simulink library "LibraryFM"  (R2016b)
settings: Solver=VariableStepAuto  StartTime=0.0  StopTime=10.0  RelTol=1e-3
undefined symbols (not defined in the file or in its folder): ActuatorStruct, drivePeakCurrent, FM1, Lb, Lf, Lu, motorTorqueConstant, RobotStruct, sampleTime, transmissionRatio
undefined symbols (not defined in the file): JointAbsoluteEncoderCounts_rev
libraries: simulink x34, LibraryFM x13, VariousBlocksLibrary x4, dspstat3 x1, simulink_extras x1, FM_Library x1
(part 1 of 3)
settings Model: Creator=niekbeckers  LastModifiedBy=Labuser

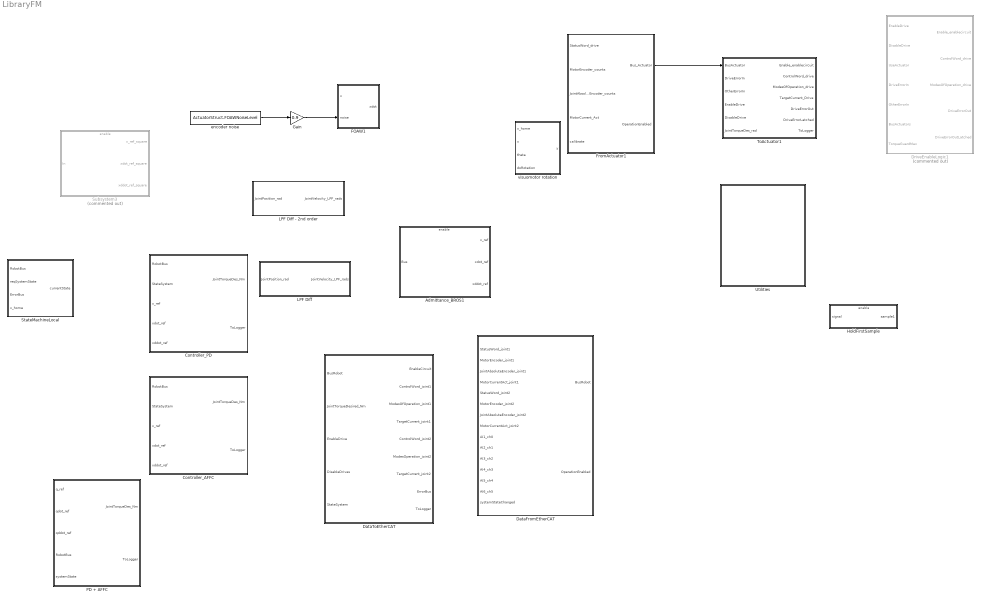
== system LibraryFM ==
  Admittance_BROS1 : Subsystem
  Controller_AFFC : Subsystem
  Controller_PD : Subsystem
  DataFromEtherCAT : Subsystem
  DataToEtherCAT : Subsystem
  DriveEnableLogic1 : Subsystem  Commented=on
  FOAW1 : MATLAB Function  TreatAsAtomicUnit=on
  FromActuator1 : Subsystem  mask{ActuatorStruct=RobotStruct.Actuator1}
      mask prompts: ActuatorStruct "Actuator Struct"
  Gain : Gain  Gain=0.9
  HoldFirstSample : Subsystem
  LPF Diff : Subsystem
  LPF Diff - 2nd order : Subsystem
  PD + AFFC : Subsystem  AncestorBlock=LibraryFM/Robot1/Controller/PD + Nonlinear ID
  StateMachineLocal : Subsystem
  Subsystem3 : Subsystem  Commented=on
  ToActuator1 : Subsystem  mask{ActuatorStruct=RobotStruct.Actuator1}
      mask prompts: ActuatorStruct "Actuator Struct"
  Utilities : Subsystem
  encoder noise : Constant  Value=ActuatorStruct.FOAWNoiseLevel
  visuomotor rotation : MATLAB Function  TreatAsAtomicUnit=on
  wires:
  FromActuator1/1(Bus_Actuator) -> ToActuator1/1(BusActuator)
  Gain/1 -> FOAW1/2(noise)
  encoder noise/1 -> Gain/1

== system LibraryFM/Admittance_BROS1 ==
  Bus : Inport
  Enable : EnablePort  StatesWhenEnabling=reset
  Bus Selector : BusSelector  OutputSignals=BusFTSensor.FxFyOpSpace
  Bus Selector1 : BusSelector  OutputSignals=xOpSpace.x_AbsEnc
  Constant : Constant
  HoldFirstSampleOnEnable : Subsystem
  Sum : Sum  Inputs=++|
  Terminator : Terminator
  Terminator1 : Terminator
  Terminator2 : Terminator
  Virtual model : MATLAB Function  TreatAsAtomicUnit=on
  virtual damping : Constant  Value=0.05
  virtual mass : Constant  Value=0.5
  x_prev : UnitDelay  SampleTime=-1
  xdot_prev : UnitDelay  SampleTime=-1
  x_ref : Outport
  xdot_ref : Outport  Port=2
  xddot_ref : Outport  Port=3
  wires:
  Virtual model/1(lim_pos) -> Terminator/1
  virtual damping/1 -> Virtual model/2(B_v)
  Sum/1 -> x_ref/1
  Virtual model/6(xddot1) -> xddot_ref/1
  x_prev/1 -> Virtual model/4(x1_prev)
  xdot_prev/1 -> Virtual model/5(xdot1_prev)
  Virtual model/5(xdot1) -> xdot_prev/1, xdot_ref/1
  Virtual model/4(x1) -> Sum/2, x_prev/1
  virtual mass/1 -> Virtual model/1(M_v)
  Virtual model/2(lim_vel) -> Terminator1/1
  Virtual model/3(lim_acc) -> Terminator2/1
  Bus/1 -> Bus Selector1/1, Bus Selector/1
  Bus Selector/1 -> Virtual model/3(F)  "<FxFyOpSpace>"
  Constant/1 -> HoldFirstSampleOnEnable/Enable
  Bus Selector1/1 -> HoldFirstSampleOnEnable/1(x)  "<x_AbsEnc>"
  HoldFirstSampleOnEnable/1(x0) -> Sum/1

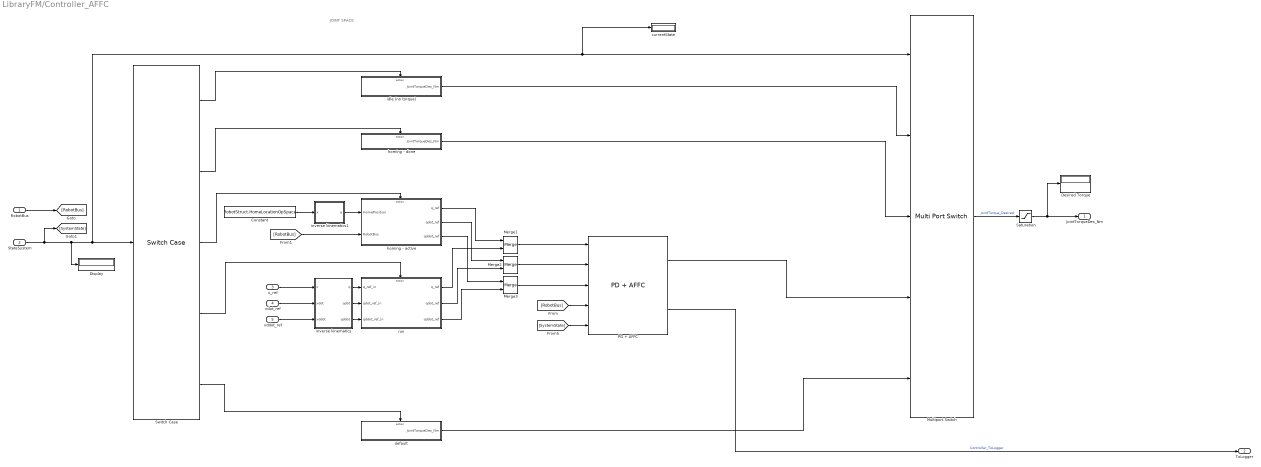
== system LibraryFM/Controller_AFFC ==
  note: JOINT SPACE
  RobotBus : Inport
  StateSystem : Inport  Port=2
  x_ref : Inport  Port=3
  xdot_ref : Inport  Port=4
  xddot_ref : Inport  Port=5
  Constant : Constant  Value=RobotStruct.HomeLocationOpSpace
  Desired Torque : Display
  Display : Display
  Merge1 : Merge  InitialOutput=[0;0]
  Merge2 : Merge  InitialOutput=[0;0]
  Merge3 : Merge  InitialOutput=[0;0]
  Multiport Switch : MultiPortSwitch  DataPortOrder=Specify indices  Inputs=4  DataPortIndices={[0,1,2,201,299,301],[399],[302,4]}  DataPortForDefault=Additional data port
  PD + AFFC : LibraryFM/PD + AFFC
  Saturation : Saturate  UpperLimit=1  LowerLimit=-2
  Switch Case : SwitchCase  CaseConditions={[0,1,2,201,299,301],[399],[302],[4]}
  currentState : Display
  default : Subsystem  TreatAsAtomicUnit=on
  homing - active : Subsystem
  homing - done : Subsystem  TreatAsAtomicUnit=on
  idle (no torque) : Subsystem  TreatAsAtomicUnit=on
  inverse kinematics : MATLAB Function  TreatAsAtomicUnit=on
  inverse kinematics1 : MATLAB Function  TreatAsAtomicUnit=on
  run : Subsystem
  JointTorqueDes_Nm : Outport
  ToLogger : Outport  Port=2
  wires:
  inverse kinematics1/1(q) -> homing - active/1(HomePosition)
  PD + AFFC/2 -> ToLogger/1  "Controller_ToLogger"
  Multiport Switch/1 -> Saturation/1  "JointTorque_Desired"
  homing - active/3(qddot_ref) -> Merge3/1
  homing - active/2(qdot_ref) -> Merge2/1
  run/3(qddot_ref) -> Merge3/2
  run/2(qdot_ref) -> Merge2/2
  StateSystem/1 -> [SystemState], Switch Case/1, currentState/1, Multiport Switch/1, Display/1
  run/1(q_ref) -> Merge1/2
  homing - active/1(q_ref) -> Merge1/1
  Switch Case/4 -> run/Action
  Saturation/1 -> JointTorqueDes_Nm/1, Desired Torque/1
  Switch Case/5 -> default/Action
  default/1(JointTorqueDes_Nm) -> Multiport Switch/5
  Switch Case/1 -> idle (no torque)/Action
  Switch Case/3 -> homing - active/Action
  Switch Case/2 -> homing - done/Action
  idle (no torque)/1(JointTorqueDes_Nm) -> Multiport Switch/2
  homing - done/1(JointTorqueDes_Nm) -> Multiport Switch/3
  Merge1/1 -> PD + AFFC/1
  Merge2/1 -> PD + AFFC/2
  Merge3/1 -> PD + AFFC/3
  PD + AFFC/1 -> Multiport Switch/4
  RobotBus/1 -> [RobotBus]
  [RobotBus] -> PD + AFFC/4
  [RobotBus] -> homing - active/2(RobotBus)
  Constant/1 -> inverse kinematics1/1(x)
  inverse kinematics/1(q) -> run/1(q_ref_in)
  inverse kinematics/2(qdot) -> run/2(qdot_ref_in)
  inverse kinematics/3(qddot) -> run/3(qddot_ref_in)
  [SystemState] -> PD + AFFC/5
  x_ref/1 -> inverse kinematics/1(x)
  xddot_ref/1 -> inverse kinematics/3(xddot)
  xdot_ref/1 -> inverse kinematics/2(xdot)

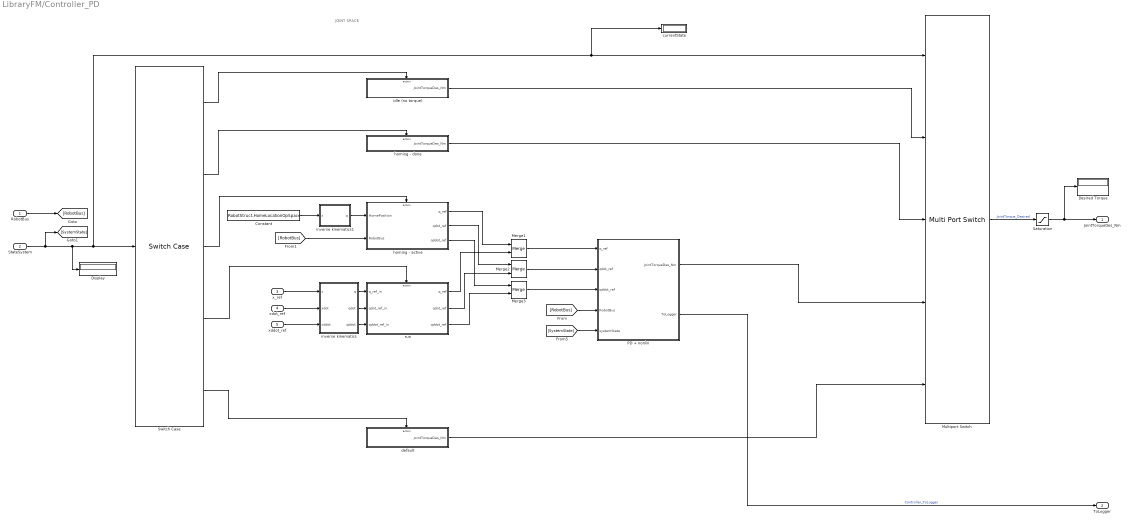
== system LibraryFM/Controller_PD ==
  note: JOINT SPACE
  RobotBus : Inport
  StateSystem : Inport  Port=2
  x_ref : Inport  Port=3
  xdot_ref : Inport  Port=4
  xddot_ref : Inport  Port=5
  Constant : Constant  Value=RobotStruct.HomeLocationOpSpace
  Desired Torque : Display
  Display : Display
  Merge1 : Merge  InitialOutput=[0;0]
  Merge2 : Merge  InitialOutput=[0;0]
  Merge3 : Merge  InitialOutput=[0;0]
  Multiport Switch : MultiPortSwitch  DataPortOrder=Specify indices  Inputs=4  DataPortIndices={[0,1,2,201,299,301],[399],[302,4]}  DataPortForDefault=Additional data port
  PD + nonlin : Subsystem
  Saturation : Saturate  UpperLimit=1  LowerLimit=-2
  Switch Case : SwitchCase  CaseConditions={[0,1,2,201,299,301],[399],[302],[4]}
  currentState : Display
  default : Subsystem  TreatAsAtomicUnit=on
  homing - active : Subsystem
  homing - done : Subsystem  TreatAsAtomicUnit=on
  idle (no torque) : Subsystem  TreatAsAtomicUnit=on
  inverse kinematics : MATLAB Function  TreatAsAtomicUnit=on
  inverse kinematics1 : MATLAB Function  TreatAsAtomicUnit=on
  run : Subsystem
  JointTorqueDes_Nm : Outport
  ToLogger : Outport  Port=2
  wires:
  inverse kinematics1/1(q) -> homing - active/1(HomePosition)
  PD + nonlin/2(ToLogger) -> ToLogger/1  "Controller_ToLogger"
  Multiport Switch/1 -> Saturation/1  "JointTorque_Desired"
  homing - active/3(qddot_ref) -> Merge3/1
  homing - active/2(qdot_ref) -> Merge2/1
  run/3(qddot_ref) -> Merge3/2
  run/2(qdot_ref) -> Merge2/2
  StateSystem/1 -> [SystemState], Switch Case/1, currentState/1, Multiport Switch/1, Display/1
  run/1(q_ref) -> Merge1/2
  homing - active/1(q_ref) -> Merge1/1
  Switch Case/4 -> run/Action
  Saturation/1 -> JointTorqueDes_Nm/1, Desired Torque/1
  Switch Case/5 -> default/Action
  default/1(JointTorqueDes_Nm) -> Multiport Switch/5
  Switch Case/1 -> idle (no torque)/Action
  Switch Case/3 -> homing - active/Action
  Switch Case/2 -> homing - done/Action
  idle (no torque)/1(JointTorqueDes_Nm) -> Multiport Switch/2
  homing - done/1(JointTorqueDes_Nm) -> Multiport Switch/3
  Merge1/1 -> PD + nonlin/1(q_ref)
  Merge2/1 -> PD + nonlin/2(qdot_ref)
  Merge3/1 -> PD + nonlin/3(qddot_ref)
  PD + nonlin/1(JointTorqueDes_Nm) -> Multiport Switch/4
  RobotBus/1 -> [RobotBus]
  [RobotBus] -> PD + nonlin/4(RobotBus)
  [RobotBus] -> homing - active/2(RobotBus)
  Constant/1 -> inverse kinematics1/1(x)
  inverse kinematics/1(q) -> run/1(q_ref_in)
  inverse kinematics/2(qdot) -> run/2(qdot_ref_in)
  inverse kinematics/3(qddot) -> run/3(qddot_ref_in)
  [SystemState] -> PD + nonlin/5(systemState)
  x_ref/1 -> inverse kinematics/1(x)
  xddot_ref/1 -> inverse kinematics/3(xddot)
  xdot_ref/1 -> inverse kinematics/2(xdot)

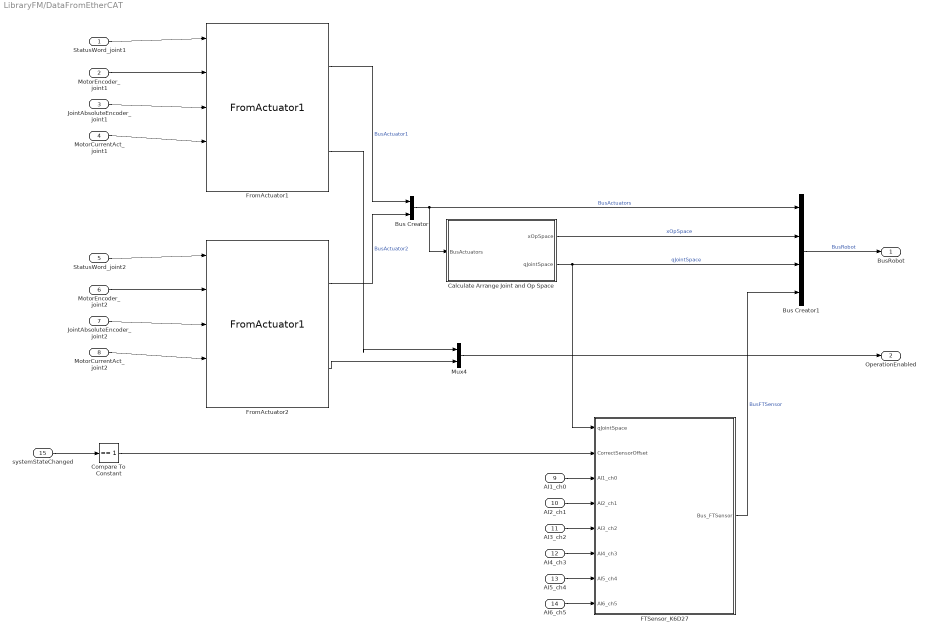
== system LibraryFM/DataFromEtherCAT ==
  StatusWord_joint1 : Inport
  MotorEncoder_joint1 : Inport  Port=2
  JointAbsoluteEncoder_joint1 : Inport  Port=3
  MotorCurrentAct_joint1 : Inport  Port=4
  StatusWord_joint2 : Inport  Port=5
  MotorEncoder_joint2 : Inport  Port=6
  "JointAbsoluteEncoder_joint2 " : Inport  Port=7
  MotorCurrentAct_joint2 : Inport  Port=8
  AI1_ch0 : Inport  Port=9
  AI2_ch1 : Inport  Port=10
  AI3_ch2 : Inport  Port=11
  AI4_ch3 : Inport  Port=12
  AI5_ch4 : Inport  Port=13
  AI6_ch5 : Inport  Port=14
  systemStateChanged : Inport  Port=15
  Bus Creator : BusCreator  Inputs=2
  Bus Creator1 : BusCreator  Inputs=4
  Calculate Arrange Joint and Op Space : Subsystem
  Compare To Constant : simulink/Logic and Bit Operations/Compare To Constant  relop===  const=1  OutDataTypeStr=boolean
  FTSensor_K6D27 : Subsystem  mask{FTSensorStruct=RobotStruct.FTSensor}
      mask prompts: FTSensorStruct "Struct for force torque sensor"
  FromActuator1 : LibraryFM/FromActuator1  ActuatorStruct=RobotStruct.Actuator1
  FromActuator2 : LibraryFM/FromActuator1  ActuatorStruct=RobotStruct.Actuator2
  Mux4 : Mux  Inputs=2
  BusRobot : Outport
  OperationEnabled : Outport  Port=2
  wires:
  Calculate Arrange Joint and Op Space/1(xOpSpace) -> Bus Creator1/2  "xOpSpace"
  Compare To Constant/1 -> FTSensor_K6D27/2(CorrectSensorOffset)
  AI6_ch5/1 -> FTSensor_K6D27/8(AI6_ch5)
  AI5_ch4/1 -> FTSensor_K6D27/7(AI5_ch4)
  AI4_ch3/1 -> FTSensor_K6D27/6(AI4_ch3)
  AI3_ch2/1 -> FTSensor_K6D27/5(AI3_ch2)
  AI2_ch1/1 -> FTSensor_K6D27/4(AI2_ch1)
  AI1_ch0/1 -> FTSensor_K6D27/3(AI1_ch0)
  systemStateChanged/1 -> Compare To Constant/1
  Calculate Arrange Joint and Op Space/2(qJointSpace) -> FTSensor_K6D27/1(qJointSpace), Bus Creator1/3  "qJointSpace"
  Bus Creator1/1 -> BusRobot/1  "BusRobot"
  Bus Creator/1 -> Bus Creator1/1, Calculate Arrange Joint and Op Space/1(BusActuators)  "BusActuators"
  MotorCurrentAct_joint2/1 -> FromActuator2/4
  "JointAbsoluteEncoder_joint2 "/1 -> FromActuator2/3
  StatusWord_joint2/1 -> FromActuator2/1
  MotorEncoder_joint2/1 -> FromActuator2/2
  MotorCurrentAct_joint1/1 -> FromActuator1/4
  JointAbsoluteEncoder_joint1/1 -> FromActuator1/3
  StatusWord_joint1/1 -> FromActuator1/1
  MotorEncoder_joint1/1 -> FromActuator1/2
  FromActuator2/2 -> Mux4/2
  Mux4/1 -> OperationEnabled/1
  FromActuator1/2 -> Mux4/1
  FromActuator2/1 -> Bus Creator/2  "BusActuator2"
  FromActuator1/1 -> Bus Creator/1  "BusActuator1"
  FTSensor_K6D27/1(Bus_FTSensor) -> Bus Creator1/4  "BusFTSensor"

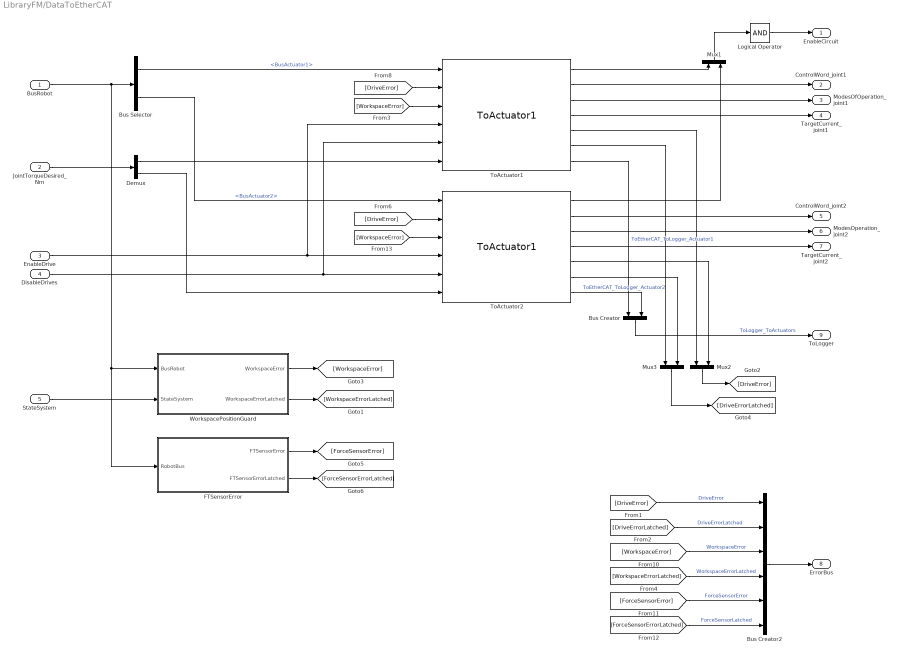
== system LibraryFM/DataToEtherCAT ==
  BusRobot : Inport
  JointTorqueDesired_Nm : Inport  Port=2
  EnableDrive : Inport  Port=3
  DisableDrives : Inport  Port=4
  StateSystem : Inport  Port=5
  Bus Creator : BusCreator  Inputs=2
  Bus Creator2 : BusCreator  Inputs=6
  Bus Selector : BusSelector  OutputSignals=BusActuators.BusActuator1,BusActuators.BusActuator2
  Demux : Demux  Outputs=2
  FTSensorError : Subsystem
  Logical Operator : Logic  Inputs=1  AllPortsSameDT=off  OutDataTypeStr=boolean
  Mux1 : Mux  Inputs=2
  Mux2 : Mux  Inputs=2
  Mux3 : Mux  Inputs=2
  ToActuator1 : LibraryFM/ToActuator1  ActuatorStruct=RobotStruct.Actuator1
  ToActuator2 : LibraryFM/ToActuator1  ActuatorStruct=RobotStruct.Actuator2
  WorkspacePositionGuard : Subsystem
  EnableCircuit : Outport  OutDataTypeStr=boolean
  ControlWord_joint1 : Outport  Port=2  OutDataTypeStr=uint16
  ModesOfOperation_joint1 : Outport  Port=3  OutDataTypeStr=int8
  TargetCurrent_joint1 : Outport  Port=4  OutDataTypeStr=int16
  ControlWord_joint2 : Outport  Port=5  OutDataTypeStr=uint16
  ModesOperation_joint2 : Outport  Port=6  OutDataTypeStr=int8
  TargetCurrent_joint2 : Outport  Port=7  OutDataTypeStr=int16
  ErrorBus : Outport  Port=8
  ToLogger : Outport  Port=9
  wires:
  WorkspacePositionGuard/2(WorkspaceErrorLatched) -> [WorkspaceErrorLatched]
  WorkspacePositionGuard/1(WorkspaceError) -> [WorkspaceError]
  FTSensorError/2(FTSensorErrorLatched) -> [ForceSensorErrorLatched]
  FTSensorError/1(FTSensorError) -> [ForceSensorError]
  [ForceSensorErrorLatched] -> Bus Creator2/6  "ForceSensorLatched"
  [ForceSensorError] -> Bus Creator2/5  "ForceSensorError"
  StateSystem/1 -> WorkspacePositionGuard/2(StateSystem)
  [WorkspaceErrorLatched] -> Bus Creator2/4  "WorkspaceErrorLatched"
  [WorkspaceError] -> Bus Creator2/3  "WorkspaceError"
  [DriveErrorLatched] -> Bus Creator2/2  "DriveErrorLatched"
  [DriveError] -> Bus Creator2/1  "DriveError"
  Bus Creator2/1 -> ErrorBus/1
  Mux3/1 -> [DriveErrorLatched]
  [WorkspaceError] -> ToActuator2/3
  [DriveError] -> ToActuator2/2
  EnableDrive/1 -> ToActuator2/4, ToActuator1/4
  DisableDrives/1 -> ToActuator2/5, ToActuator1/5
  [WorkspaceError] -> ToActuator1/3
  Bus Selector/1 -> ToActuator1/1  "<BusActuator1>"
  Bus Selector/2 -> ToActuator2/1  "<BusActuator2>"
  BusRobot/1 -> Bus Selector/1, FTSensorError/1(RobotBus), WorkspacePositionGuard/1(BusRobot)
  Demux/1 -> ToActuator1/6
  JointTorqueDesired_Nm/1 -> Demux/1
  Demux/2 -> ToActuator2/6
  Logical Operator/1 -> EnableCircuit/1
  ToActuator2/3 -> ModesOperation_joint2/1
  ToActuator2/4 -> TargetCurrent_joint2/1
  ToActuator1/4 -> TargetCurrent_joint1/1
  ToActuator2/2 -> ControlWord_joint2/1
  ToActuator1/3 -> ModesOfOperation_joint1/1
  ToActuator1/2 -> ControlWord_joint1/1
  ToActuator2/1 -> Mux1/2
  ToActuator1/1 -> Mux1/1
  Mux1/1 -> Logical Operator/1
  [DriveError] -> ToActuator1/2
  ToActuator2/6 -> Mux3/2
  ToActuator1/6 -> Mux3/1
  Mux2/1 -> [DriveError]
  ToActuator2/5 -> Mux2/2
  ToActuator1/5 -> Mux2/1
  ToActuator1/7 -> Bus Creator/1  "ToEtherCAT_ToLogger_Actuator1"
  ToActuator2/7 -> Bus Creator/2  "ToEtherCAT_ToLogger_Actuator2"
  Bus Creator/1 -> ToLogger/1  "ToLogger_ToActuators"

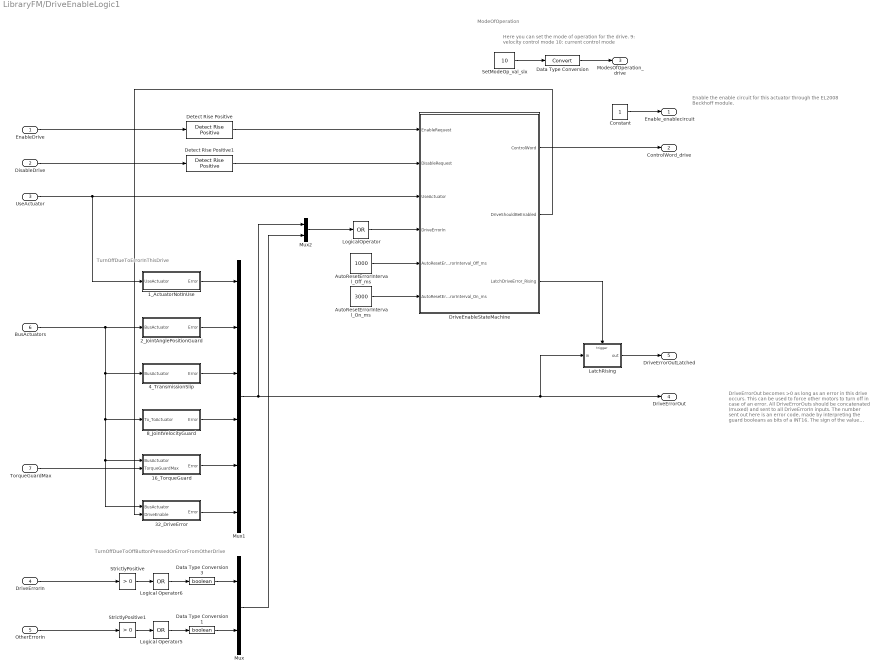
== system LibraryFM/DriveEnableLogic1 ==
  note: Here you can set the mode of operation for the drive.
      | 9: velocity control mode
      | 10: current control mode
  note: TurnOffDueToErrorInThisDrive
  note: TurnOffDueToOffButtonPressedOrErrorFromOtherDrive
  note: DriveErrorOut becomes >0 as long as an error in this drive occurs. This can be used to force other motors to turn off in case of an error.
      | All DriveErrorOuts should be concatenated (muxed)  and sent to all DriveErrorIn inputs. The number sent out here is an error code, made by interpreting the guard booleans as bits of a INT16.
      | The sign of the value indicates:
      | >=0: UseActuator=true
      | <0: UseActuator = False
  note: ModeOfOperation
  note: Enable the enable circuit for this actuator through the EL2008
      | Beckhoff module.
  EnableDrive : Inport
  DisableDrive : Inport  Port=2
  UseActuator : Inport  Port=3
  DriveErrorIn : Inport  Port=4
  OtherErrorIn : Inport  Port=5
  BusActuators : Inport  Port=6
  TorqueGuardMax : Inport  Port=7
  16_TorqueGuard : Subsystem
  1_ActuatorNotInUse : Subsystem
  2_JointAnglePositionGuard : Subsystem
  32_DriveError : Subsystem
  4_TransmissionSlip : Subsystem
  8_JointVelocityGuard : Subsystem
  AutoResetErrorInterval_Off_ms : Constant  Value=1000
  AutoResetErrorInterval_On_ms : Constant  Value=3000
  Constant : Constant
  Data Type Conversion : DataTypeConversion
  Data Type Conversion1 : DataTypeConversion  OutDataTypeStr=boolean
  Data Type Conversion3 : DataTypeConversion  OutDataTypeStr=boolean
  Detect Rise Positive : simulink/Logic and Bit Operations/Detect Rise Positive  vinit=0  InputProcessing=Inherited  OutDataTypeStr=boolean
  Detect Rise Positive1 : simulink/Logic and Bit Operations/Detect Rise Positive  vinit=0  InputProcessing=Inherited  OutDataTypeStr=boolean
  DriveEnableStateMachine : Stateflow chart  TreatAsAtomicUnit=on
  LatchRising : Subsystem  TreatAsAtomicUnit=on
  Logical Operator5 : Logic  Operator=OR  Inputs=1  AllPortsSameDT=off  OutDataTypeStr=boolean
  Logical Operator6 : Logic  Operator=OR  Inputs=1  AllPortsSameDT=off  OutDataTypeStr=boolean
  LogicalOperator : Logic  Operator=OR  Inputs=1  AllPortsSameDT=off  OutDataTypeStr=boolean
  Mux : Mux  Inputs=2
  Mux1 : Mux  Inputs=6
  Mux2 : Mux  Inputs=2
  SetModeOp_val_slx : Constant  Value=10
  StrictlyPositive : simulink/Logic and Bit Operations/Compare To Zero  relop=>  OutDataTypeStr=boolean
  StrictlyPositive1 : simulink/Logic and Bit Operations/Compare To Zero  relop=>  OutDataTypeStr=boolean
  Enable_enablecircuit : Outport
  ControlWord_drive : Outport  Port=2
  ModesOfOperation_drive : Outport  Port=3
  DriveErrorOut : Outport  Port=4
  DriveErrorOutLatched : Outport  Port=5
  wires:
  OtherErrorIn/1 -> StrictlyPositive1/1
  Logical Operator5/1 -> Data Type Conversion1/1
  Data Type Conversion3/1 -> Mux/1
  16_TorqueGuard/1(Error) -> Mux1/5
  32_DriveError/1(Error) -> Mux1/6
  1_ActuatorNotInUse/1(Error) -> Mux1/1
  BusActuators/1 -> 4_TransmissionSlip/1(BusActuator), 8_JointVelocityGuard/1(To_ToActuator), 32_DriveError/1(BusActuator), 16_TorqueGuard/1(BusActuator), 2_JointAnglePositionGuard/1(BusActuator)
  Mux/1 -> Mux2/2
  Logical Operator6/1 -> Data Type Conversion3/1
  DriveErrorIn/1 -> StrictlyPositive/1
  UseActuator/1 -> 1_ActuatorNotInUse/1(UseActuator), DriveEnableStateMachine/3(UseActuator)
  Data Type Conversion/1 -> ModesOfOperation_drive/1
  DisableDrive/1 -> Detect Rise Positive1/1
  EnableDrive/1 -> Detect Rise Positive/1
  SetModeOp_val_slx/1 -> Data Type Conversion/1
  TorqueGuardMax/1 -> 16_TorqueGuard/2(TorqueGuardMax)
  StrictlyPositive/1 -> Logical Operator6/1
  Mux1/1 -> DriveErrorOut/1, LatchRising/1(in), Mux2/1
  4_TransmissionSlip/1(Error) -> Mux1/3
  2_JointAnglePositionGuard/1(Error) -> Mux1/2
  LatchRising/1(out) -> DriveErrorOutLatched/1
  8_JointVelocityGuard/1(Error) -> Mux1/4
  StrictlyPositive1/1 -> Logical Operator5/1
  Data Type Conversion1/1 -> Mux/2
  AutoResetErrorInterval_Off_ms/1 -> DriveEnableStateMachine/5(AutoResetErrorInterval_Off_ms)
  AutoResetErrorInterval_On_ms/1 -> DriveEnableStateMachine/6(AutoResetErrorInterval_On_ms)
  LogicalOperator/1 -> DriveEnableStateMachine/4(DriveErrorIn)
  Detect Rise Positive1/1 -> DriveEnableStateMachine/2(DisableRequest)
  Detect Rise Positive/1 -> DriveEnableStateMachine/1(EnableRequest)
  DriveEnableStateMachine/1(ControlWord) -> ControlWord_drive/1
  DriveEnableStateMachine/2(DriveShouldBeEnabled) -> 32_DriveError/2(DriveEnable)
  Mux2/1 -> LogicalOperator/1
  DriveEnableStateMachine/3(LatchDriveError_Rising) -> LatchRising/Trigger
  Constant/1 -> Enable_enablecircuit/1

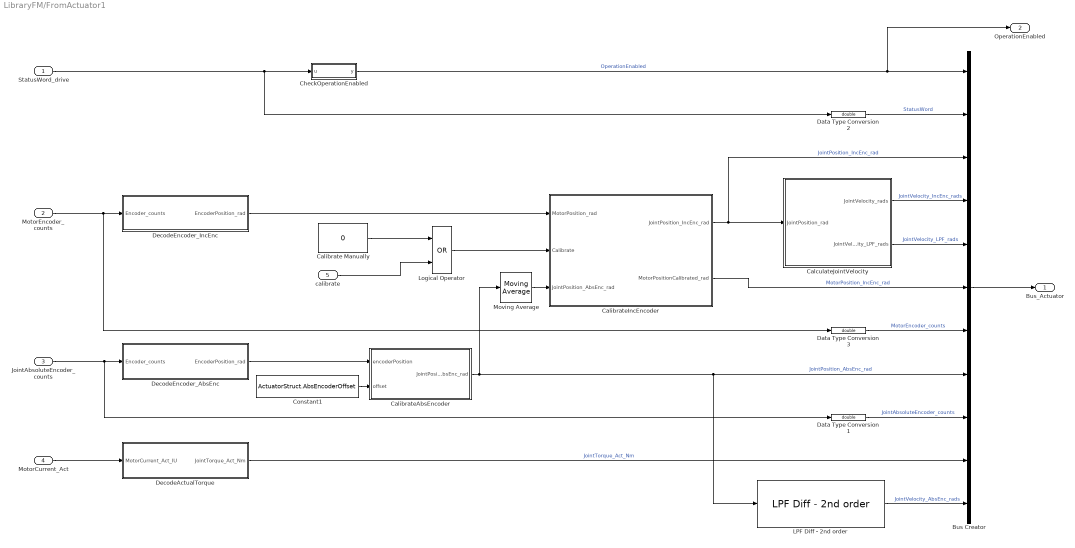
== system LibraryFM/FromActuator1 ==
  StatusWord_drive : Inport
  MotorEncoder_counts : Inport  Port=2
  JointAbsoluteEncoder_counts : Inport  Port=3
  MotorCurrent_Act : Inport  Port=4
  calibrate : Inport  Port=5
  Bus Creator : BusCreator  Inputs=11
  CalculateJointVelocity : Subsystem
  Calibrate Manually : Constant  Value=0
      settings: OpenFcn=set_param(gcb,'Value','1');tname = ['toggletimer_' gcb];delete(timerfind('name',tname));t = timer('timerfcn', ['set_param(''',gcb,''',''Value'',''0'')'],'executionmode','singleshot','startdelay',1,'name',tname);start(t);
      mask Display: fprintf('PushToTrigger\n%s',get_param(gcb,'value'))
  CalibrateAbsEncoder : MATLAB Function  TreatAsAtomicUnit=on
  "CalibrateIncEncoder    " : MATLAB Function  TreatAsAtomicUnit=on  mask{transmissionRatio=ActuatorStruct.transmissionRatio}
      mask prompts: transmissionRatio "Transmission ratio (e.g. -8) [-]"
  CheckOperationEnabled : MATLAB Function  TreatAsAtomicUnit=on
  Constant1 : Constant  Value=ActuatorStruct.AbsEncoderOffset
  Data Type Conversion1 : DataTypeConversion  OutDataTypeStr=double
  Data Type Conversion2 : DataTypeConversion  OutDataTypeStr=double
  Data Type Conversion3 : DataTypeConversion  OutDataTypeStr=double
  DecodeActualTorque : MATLAB Function  TreatAsAtomicUnit=on  mask(DecodeActualTorque){transmissionRatio=ActuatorStruct.transmissionRatio, motorTorqueConstant=ActuatorStruct.motorTorqueConstant, drivePeakCurrent=ActuatorStruct.drivePeakCurrent}
      mask prompts: transmissionRatio "Transmission ratio (e.g. -8) [-]"; motorTorqueConstant "Motor torque constant [Nm/A]"; drivePeakCurrent "Motor drive peak current Ipeak [A]"
      mask help:
      | Decode Actual Torque value returned from the actuator (motor drive and motor) to torque on the joint (after transmission).
      |
      | Note: due to the way the transmission is set up and the positive motor axis (clockwise is positive as seen from the motor front), there is no need to account for sign change in motor torque or encoder position.
  DecodeEncoder_AbsEnc : MATLAB Function  TreatAsAtomicUnit=on  mask(DecodeEncoder){EncoderCounts_rev=ActuatorStruct.JointAbsoluteEncoderCounts_rev}
      mask prompts: EncoderCounts_rev "Motor encoder increments per revolution (e.g., 8192)"
      mask help: Decode the encoder counts to encoder position in radians
  DecodeEncoder_IncEnc : MATLAB Function  TreatAsAtomicUnit=on  mask(DecodeEncoder){EncoderCounts_rev=ActuatorStruct.MotorEncoderCounts_rev}
      mask prompts: EncoderCounts_rev "Motor encoder increments per revolution (e.g., 8192)"
      mask help: Decode the encoder counts to encoder position in radians
  LPF Diff - 2nd order : LibraryFM/LPF Diff - 2nd order
  Logical Operator : Logic  Operator=OR  AllPortsSameDT=off  OutDataTypeStr=boolean
  Moving Average : dspstat3/Moving Average  Method=Sliding window  SpecifyWindowLength=on  WindowLength=500  ForgettingFactor=0.9  SimulateUsing=Code generation
  Bus_Actuator : Outport
  OperationEnabled : Outport  Port=2
  wires:
  calibrate/1 -> Logical Operator/2
  Logical Operator/1 -> "CalibrateIncEncoder    "/2(Calibrate)
  Calibrate Manually/1 -> Logical Operator/1
  Constant1/1 -> CalibrateAbsEncoder/2(offset)
  Bus Creator/1 -> Bus_Actuator/1
  Data Type Conversion3/1 -> Bus Creator/7  "MotorEncoder_counts"
  MotorEncoder_counts/1 -> Data Type Conversion3/1, DecodeEncoder_IncEnc/1(Encoder_counts)
  CalibrateAbsEncoder/1(JointPosition_AbsEnc_rad) -> Moving Average/1, LPF Diff - 2nd order/1, Bus Creator/8  "JointPosition_AbsEnc_rad"
  Data Type Conversion2/1 -> Bus Creator/2  "StatusWord"
  Data Type Conversion1/1 -> Bus Creator/9  "JointAbsoluteEncoder_counts"
  "CalibrateIncEncoder    "/1(JointPosition_IncEnc_rad) -> Bus Creator/3, CalculateJointVelocity/1(JointPosition_rad)  "JointPosition_IncEnc_rad"
  JointAbsoluteEncoder_counts/1 -> DecodeEncoder_AbsEnc/1(Encoder_counts), Data Type Conversion1/1
  CheckOperationEnabled/1(y) -> Bus Creator/1, OperationEnabled/1  "OperationEnabled"
  MotorCurrent_Act/1 -> DecodeActualTorque/1(MotorCurrent_Act_IU)
  DecodeEncoder_IncEnc/1(EncoderPosition_rad) -> "CalibrateIncEncoder    "/1(MotorPosition_rad)
  StatusWord_drive/1 -> Data Type Conversion2/1, CheckOperationEnabled/1(u)
  DecodeActualTorque/1(JointTorque_Act_Nm) -> Bus Creator/10  "JointTorque_Act_Nm"
  "CalibrateIncEncoder    "/2(MotorPositionCalibrated_rad) -> Bus Creator/6  "MotorPosition_IncEnc_rad"
  DecodeEncoder_AbsEnc/1(EncoderPosition_rad) -> CalibrateAbsEncoder/1(encoderPosition)
  CalculateJointVelocity/1(JointVelocity_rads) -> Bus Creator/4  "JointVelocity_IncEnc_rads"
  Moving Average/1 -> "CalibrateIncEncoder    "/3(JointPosition_AbsEnc_rad)
  CalculateJointVelocity/2(JointVelocity_LPF_rads) -> Bus Creator/5  "JointVelocity_LPF_rads"
  LPF Diff - 2nd order/1 -> Bus Creator/11  "JointVelocity_AbsEnc_rads"

== system LibraryFM/HoldFirstSample ==
  note: These blocks hold the first sample of the input
      | when the block is enabled (through the action port)
  signal : Inport
  Enable : EnablePort
  Counter Free-Running : simulink/Sources/Counter Free-Running  NumBits=32  tsamp=-1
  Memory1 : Memory
  Switch : Switch  Threshold=1
  sample1 : Outport
  wires:
  signal/1 -> Switch/3
  Memory1/1 -> Switch/1
  Switch/1 -> sample1/1, Memory1/1
  Counter Free-Running/1 -> Switch/2

== system LibraryFM/LPF Diff ==
  JointPosition_rad : Inport
  Discrete Derivative : simulink/Discrete/Discrete Derivative  gainval=1.0  ICPrevScaledInput=0.0  InputProcessing=Inherited  OutMin=[]  OutMax=[]  OutDataType=fixdt(1, 16)  OutScaling=2^-10  DoSatur=off
  Freq [Hz] : Constant  Value=200  OutDataTypeStr=double
  MATLAB Function : MATLAB Function  TreatAsAtomicUnit=on
  Unit Delay : UnitDelay  SampleTime=-1
  JointVelocity_LPF_rads : Outport
  wires:
  Discrete Derivative/1 -> MATLAB Function/1(u)
  MATLAB Function/1(y) -> JointVelocity_LPF_rads/1, Unit Delay/1
  JointPosition_rad/1 -> Discrete Derivative/1
  Unit Delay/1 -> MATLAB Function/3(y_prev)
  Freq [Hz]/1 -> MATLAB Function/2(freq)

== system LibraryFM/LPF Diff - 2nd order ==
  JointPosition_rad : Inport
  Butterworth filter : DiscreteFilter  Numerator=ActuatorStruct.FilterButterB  Denominator=ActuatorStruct.FilterButterA  FilterStructure=Direct form I
  Discrete Derivative : simulink/Discrete/Discrete Derivative  gainval=1.0  ICPrevScaledInput=0.0  InputProcessing=Inherited  OutMin=[]  OutMax=[]  OutDataType=fixdt(1, 16)  OutScaling=2^-10  DoSatur=off
  JointVelocity_LPF_rads : Outport
  wires:
  JointPosition_rad/1 -> Discrete Derivative/1
  Discrete Derivative/1 -> Butterworth filter/1
  Butterworth filter/1 -> JointVelocity_LPF_rads/1

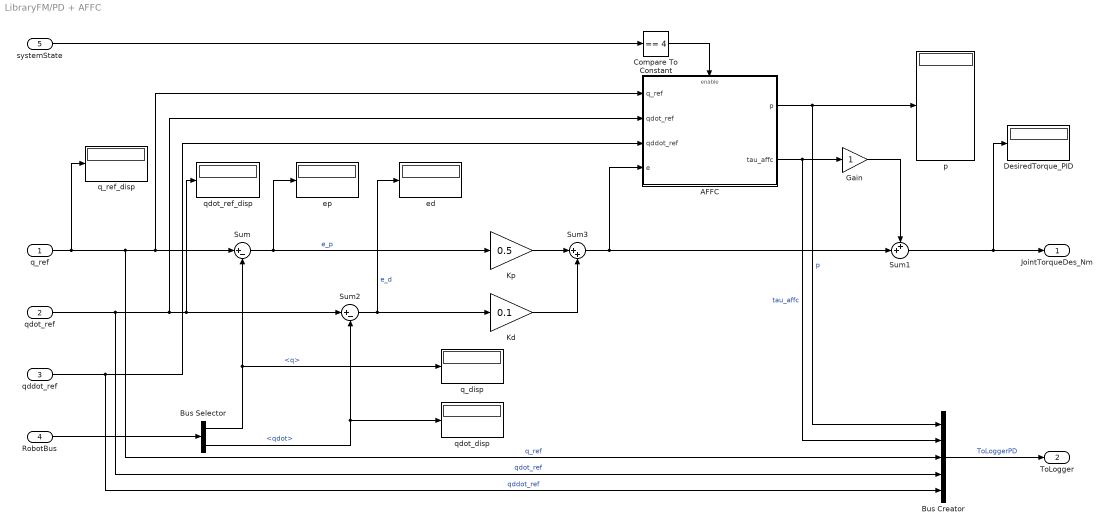
== system LibraryFM/PD + AFFC ==
  q_ref : Inport
  qdot_ref : Inport  Port=2
  qddot_ref : Inport  Port=3
  RobotBus : Inport  Port=4
  systemState : Inport  Port=5
  AFFC : Subsystem
  Bus Creator : BusCreator  Inputs=5
  Bus Selector : BusSelector  OutputSignals=qJointSpace.q,qJointSpace.qdot
  Compare To Constant : simulink/Logic and Bit Operations/Compare To Constant  relop===  const=4  OutDataTypeStr=boolean
  DesiredTorque_PID : Display
  Gain : Gain
  Kd : Gain  Gain=0.1
  Kp : Gain  Gain=0.5
  Sum : Sum  Inputs=|+-
  Sum1 : Sum  Inputs=++|
  Sum2 : Sum  Inputs=|+-
  Sum3 : Sum  Inputs=|++
  ed : Display
  ep : Display
  p : Display
  q_disp : Display
  q_ref_disp : Display
  qdot_disp : Display
  qdot_ref_disp : Display
  JointTorqueDes_Nm : Outport
  ToLogger : Outport  Port=2
  wires:
  Bus Selector/2 -> Sum2/2, qdot_disp/1  "<qdot>"
  Bus Selector/1 -> Sum/2, q_disp/1  "<q>"
  q_ref/1 -> Bus Creator/3, AFFC/1(q_ref), Sum/1, q_ref_disp/1  "q_ref"
  Sum/1 -> Kp/1, ep/1  "e_p"
  Sum3/1 -> AFFC/4(e), Sum1/2
  Kd/1 -> Sum3/2
  Kp/1 -> Sum3/1
  qdot_ref/1 -> Bus Creator/4, AFFC/2(qdot_ref), Sum2/1, qdot_ref_disp/1  "qdot_ref"
  Sum2/1 -> Kd/1, ed/1  "e_d"
  Gain/1 -> Sum1/1
  Sum1/1 -> JointTorqueDes_Nm/1, DesiredTorque_PID/1
  RobotBus/1 -> Bus Selector/1
  qddot_ref/1 -> Bus Creator/5, AFFC/3(qddot_ref)  "qddot_ref"
  AFFC/1(p) -> Bus Creator/1, p/1  "p"
  AFFC/2(tau_affc) -> Bus Creator/2, Gain/1  "tau_affc"
  systemState/1 -> Compare To Constant/1
  Compare To Constant/1 -> AFFC/Enable
  Bus Creator/1 -> ToLogger/1  "ToLoggerPD"

== system LibraryFM/StateMachineLocal ==
  note: Very crude error handling
      | Ideally, the state machine gets all
      | the error codes (2,4,8, etc) such that
      | it can discern between states
  RobotBus : Inport
  reqSystemState : Inport  Port=2
  ErrorBus : Inport  Port=3
  x_home : Inport  Port=4
  Bus Selector : BusSelector  OutputSignals=qJointSpace.qdot_IncEnc,xOpSpace.x
  Bus Selector1 : BusSelector  OutputSignals=ErrorCode  OutputAsBus=on
  CheckVelThreshold : MATLAB Function  TreatAsAtomicUnit=on
  Compare To Constant : simulink/Logic and Bit Operations/Compare To Constant  relop=>  const=0  OutDataTypeStr=boolean
  Constant : Constant  Value=RobotStruct.HomeLocationSize
  Constant2 : Constant  Value=0.05
  Detect Change1 : simulink/Logic and Bit Operations/Detect Change  Commented=on  vinit=0  InputProcessing=Inherited  OutDataTypeStr=boolean
  Encode system state change : MATLAB Function  Commented=on  TreatAsAtomicUnit=on
  Logical Operator : Logic  Operator=OR  Inputs=1  AllPortsSameDT=off  OutDataTypeStr=boolean
  State machine : Stateflow chart  TreatAsAtomicUnit=on
  Terminator : Terminator  Commented=on
  checkEndpointPosition : MATLAB Function  TreatAsAtomicUnit=on
  system state : Display
  currentState : Outport
  wires:
  Bus Selector1/1 -> Compare To Constant/1
  ErrorBus/1 -> Bus Selector1/1
  State machine/1(currentState) -> currentState/1, system state/1
  Logical Operator/1 -> State machine/2(fault)
  Compare To Constant/1 -> Logical Operator/1
  reqSystemState/1 -> State machine/1(requestedState)
  Detect Change1/1 -> Encode system state change/1(stateChanged)
  Encode system state change/1(systemStateChanged) -> Terminator/1
  RobotBus/1 -> Bus Selector/1
  Bus Selector/1 -> CheckVelThreshold/1(qdot)  "<qdot_IncEnc>"
  Bus Selector/2 -> checkEndpointPosition/1(x)  "<x>"
  CheckVelThreshold/1(velBelowThreshold) -> State machine/3(velBelowThreshold)
  Constant2/1 -> CheckVelThreshold/2(threshold)
  x_home/1 -> checkEndpointPosition/2(homeLocation)
  Constant/1 -> checkEndpointPosition/3(threshold)
  checkEndpointPosition/1(isAtEndpoint) -> State machine/4(isAtHome)

== system LibraryFM/Subsystem3 ==
  In : Inport
  Enable : EnablePort  StatesWhenEnabling=reset
  Constant : Constant  Value=[0;0]
  Sum2 : Sum  Inputs=++|
  Terminator : Terminator
  pos_boundary : Constant  Value=0.065
  prev_x : UnitDelay  InitialCondition=[0;0]  SampleTime=-1
  vel : Constant  Value=0.15
  virtual mass2 : Constant  Value=FM1.HomeLocationOpSpace
  visuomotor rotation1 : MATLAB Function  TreatAsAtomicUnit=on
  x_ref_square : Outport  InitialOutput=[0;0]
  xdot_ref_square : Outport  Port=2  InitialOutput=[0;0]
  xddot_ref_square : Outport  Port=3  InitialOutput=[0;0]
  wires:
  vel/1 -> visuomotor rotation1/3(vel)
  pos_boundary/1 -> visuomotor rotation1/2(yBound), visuomotor rotation1/1(xBound)
  visuomotor rotation1/1(pos_ref) -> Sum2/2, prev_x/1
  prev_x/1 -> visuomotor rotation1/4(pos_ref_prev)
  visuomotor rotation1/2(vel_ref) -> xdot_ref_square/1
  virtual mass2/1 -> Sum2/1
  Sum2/1 -> x_ref_square/1
  Constant/1 -> xddot_ref_square/1
  In/1 -> Terminator/1

== system LibraryFM/ToActuator1 ==
  note: The Latched version keeps the most recent value from when the motor was on; in other words, the reason why the motor turned off.
  note: The UseActuator block can be used to enable or disable the actuator altogether.
  BusActuator : Inport
  DriveErrorIn : Inport  Port=2
  OtherErrorIn : Inport  Port=3
  EnableDrive : Inport  Port=4
  DisableDrive : Inport  Port=5
  JointTorqueDes_rad : Inport  Port=6
  AppendToBus : Subsystem
  DriveEnableLogic : Subsystem
  EncodeDesiredTorque : MATLAB Function  TreatAsAtomicUnit=on  mask(EncodeDesiredTorque){transmissionRatio=ActuatorStruct.transmissionRatio, motorTorqueConstant=ActuatorStruct.motorTorqueConstant, drivePeakCurrent=ActuatorStruct.drivePeakCurrent}
      mask prompts: transmissionRatio "Transmission ratio (e.g. -8) [-]"; motorTorqueConstant "Motor torque constant [Nm/A]"; drivePeakCurrent "Motor drive peak current [A]"
      mask help:
      | Encode desired torque at the joint to torque to be produced by the motor.
      |
      | Note: due to the way the transmission is set up and the positive motor axis (clockwise is positive as seen from the motor front), there is no need to account for sign change in motor torque or encoder position.
  PreventAlgebraicLoop : Memory
  TorqueLimit_Nm : Constant  Value=ActuatorStruct.AbsoluteMaximumTorque_Nm
  TorqueLimiter : LibraryFM/Utilities/TorqueLimiter
  UseActuator : Constant  OutDataTypeStr=double
      settings: OpenFcn=|
      | b = get_param(gcb,'value');
      | if (strcmp(b,'1')),
      |   set_param (gcb,'value','0');
      | else
      |   set_param(gcb,'value','1');
      | end;
  Enable_enablecircuit : Outport
  ControlWord_drive : Outport  Port=2
  ModesOfOperation_drive : Outport  Port=3
  TargetCurrent_Drive : Outport  Port=4
  DriveErrorOut : Outport  Port=5
  DriveErrorLatched : Outport  Port=6
  ToLogger : Outport  Port=7
  wires:
  OtherErrorIn/1 -> DriveEnableLogic/5(OtherErrorIn)
  DriveEnableLogic/1(Enable_enablecircuit) -> Enable_enablecircuit/1
  JointTorqueDes_rad/1 -> TorqueLimiter/2, AppendToBus/3(DesiredTorque)
  TorqueLimiter/1 -> DriveEnableLogic/7(TorqueGuardMax)
  TorqueLimiter/2 -> AppendToBus/4(DesiredTorqueLimited), EncodeDesiredTorque/1(JointTorque_Des_Nm)
  DriveEnableLogic/5(DriveErrorOutLatched) -> DriveErrorLatched/1
  TorqueLimit_Nm/1 -> TorqueLimiter/1
  DriveEnableLogic/3(ModesOfOperation_drive) -> ModesOfOperation_drive/1
  DriveEnableLogic/2(ControlWord_drive) -> ControlWord_drive/1
  EncodeDesiredTorque/1(MotorTorque_Des_IU) -> TargetCurrent_Drive/1
  BusActuator/1 -> DriveEnableLogic/6(BusActuators), AppendToBus/1(Bus_in)
  EnableDrive/1 -> DriveEnableLogic/1(EnableDrive)
  DisableDrive/1 -> DriveEnableLogic/2(DisableDrive)
  DriveErrorIn/1 -> DriveEnableLogic/4(DriveErrorIn)
  AppendToBus/1(Bus_out) -> ToLogger/1
  UseActuator/1 -> DriveEnableLogic/3(UseActuator)
  DriveEnableLogic/4(DriveErrorOut) -> PreventAlgebraicLoop/1, AppendToBus/2(DriveError)
  PreventAlgebraicLoop/1 -> DriveErrorOut/1

== system LibraryFM/Utilities ==
  Boolean : Constant  Value=false  OutDataTypeStr=boolean
      settings: OpenFcn=|
      | b = get_param(gcb,'value');
      | if (strcmp(b,'true')),
      |   set_param (gcb,'value','false');
      | else
      |   set_param(gcb,'value','true');
      | end;
  Boolean1 : Constant  OutDataTypeStr=double
      settings: OpenFcn=|
      | b = get_param(gcb,'value');
      | if (strcmp(b,'1')),
      |   set_param (gcb,'value','0');
      | else
      |   set_param(gcb,'value','1');
      | end;
  CrossFade : Subsystem
  Cycloid : Subsystem
  DecodeActualTorque : MATLAB Function  TreatAsAtomicUnit=on  mask(DecodeActualTorque){transmissionRatio=transmissionRatio, motorTorqueConstant=motorTorqueConstant, drivePeakCurrent=drivePeakCurrent}
      mask prompts: transmissionRatio "Transmission ratio (e.g. -8) [-]"; motorTorqueConstant "Motor torque constant [Nm/A]"; drivePeakCurrent "Motor drive peak current Ipeak [A]"
      mask help:
      | Decode Actual Torque value returned from the actuator (motor drive and motor) to torque on the joint (after transmission).
      |
      | Note: due to the way the transmission is set up and the positive motor axis (clockwise is positive as seen from the motor front), there is no need to account for sign change in motor torque or encoder position.
  DecodeEncoder : MATLAB Function  TreatAsAtomicUnit=on  mask(DecodeEncoder){EncoderCounts_rev=JointAbsoluteEncoderCounts_rev}
      mask prompts: EncoderCounts_rev "Motor encoder increments per revolution (e.g., 8192)"
      mask help: Decode the encoder counts to encoder position in radians
  EncodeDesiredTorque : MATLAB Function  TreatAsAtomicUnit=on  mask(EncodeDesiredTorque){transmissionRatio=transmissionRatio, motorTorqueConstant=motorTorqueConstant, drivePeakCurrent=drivePeakCurrent}
      mask prompts: transmissionRatio "Transmission ratio (e.g. -8) [-]"; motorTorqueConstant "Motor torque constant [Nm/A]"; drivePeakCurrent "Motor drive peak current [A]"
      mask help:
      | Encode desired torque at the joint to torque to be produced by the motor.
      |
      | Note: due to the way the transmission is set up and the positive motor axis (clockwise is positive as seen from the motor front), there is no need to account for sign change in motor torque or encoder position.
  EndstopAndSafety : Subsystem
  FOAW : MATLAB Function  TreatAsAtomicUnit=on
  FilterFourthOrder : Subsystem
  Latch : Subsystem  mask{ic=0}
      mask prompts: ic "Initial Condition"
  LatchRising : Subsystem  mask{ic=0}
      mask prompts: ic "Initial Condition"
  MonoStable : Constant  Value=0
      settings: OpenFcn=|
      | set_param(gcb,'Value','1');
      | tname = ['toggletimer_' gcb];
      | delete(timerfind('name',tname));
      | t = timer('timerfcn', ['set_param(''',gcb,''',''Value'',''0'')'],'executionmode','singleshot','startdelay',1,'name',tname);
      | start(t);
      mask Display: fprintf('PushToTrigger\n%s',get_param(gcb,'value'))
  Stopwatch : Subsystem
  TorqueLimiter : Subsystem

== system LibraryFM/Admittance_BROS1/HoldFirstSampleOnEnable ==
  note: These blocks hold the first sample of the input
      | when the block is enabled (through the action port)
  x : Inport
  Enable : EnablePort  StatesWhenEnabling=reset
  Counter Free-Running : simulink/Sources/Counter Free-Running  NumBits=32  tsamp=-1
  Display : Display
  Memory1 : Memory
  Switch : Switch  Threshold=1
  x0 : Outport
  wires:
  x/1 -> Switch/3
  Counter Free-Running/1 -> Switch/2
  Memory1/1 -> Switch/1
  Switch/1 -> x0/1, Memory1/1, Display/1

== system LibraryFM/Controller_AFFC/default ==
  Action Port : ActionPort  InitializeStates=reset
  Constant3 : Constant  Value=[0;0]
  JointTorqueDes_Nm : Outport  InitialOutput=[0;0]
  wires:
  Constant3/1 -> JointTorqueDes_Nm/1

== system LibraryFM/Controller_AFFC/homing - active ==
  note: The velocity and acceleration references are set to [0;0] for stability.
  note: These blocks hold the first sample of the input
      | when the block is enabled (through the action port)
  HomePosition : Inport
  RobotBus : Inport  Port=2
  Action Port : ActionPort  InitializeStates=reset
  Bus Selector : BusSelector  OutputSignals=qJointSpace.q
  Constant1 : Constant
  Constant2 : Constant  Value=[0;0]
  Constant4 : Constant  Value=[0;0]
  Counter Free-Running : simulink/Sources/Counter Free-Running  NumBits=32  tsamp=-1
  CrossFade : VariousBlocksLibrary/Various/CrossFade
  Cycloid : VariousBlocksLibrary/Various/Cycloid
  Manual Switch : ManualSwitch  CurrentSetting=0
  Memory1 : Memory
  Rate Limiter : RateLimiter  RisingSlewLimit=0.1  FallingSlewLimit=-0.2  SampleTimeMode=inherited
  Switch : Switch  Threshold=1
  q_ref : Outport  InitialOutput=[0;0]
  qdot_ref : Outport  Port=2  InitialOutput=[0;0]
  qddot_ref : Outport  Port=3  InitialOutput=[0;0]
  wires:
  Constant4/1 -> qddot_ref/1
  CrossFade/1 -> q_ref/1
  Manual Switch/1 -> CrossFade/1
  Memory1/1 -> Switch/1
  Counter Free-Running/1 -> Switch/2
  Switch/1 -> Manual Switch/1, Memory1/1
  Constant1/1 -> Rate Limiter/1
  Rate Limiter/1 -> Cycloid/1
  Cycloid/1 -> CrossFade/3
  HomePosition/1 -> CrossFade/2
  RobotBus/1 -> Bus Selector/1
  Bus Selector/1 -> Switch/3, Manual Switch/2  "<q>"
  Constant2/1 -> qdot_ref/1

== system LibraryFM/Controller_AFFC/homing - done ==
  Action Port : ActionPort
  Constant : Constant  Value=[0;0]
  JointTorqueDes_Nm : Outport  InitialOutput=[0;0]
  wires:
  Constant/1 -> JointTorqueDes_Nm/1

== system LibraryFM/Controller_AFFC/idle (no torque) ==
  Action Port : ActionPort  InitializeStates=reset
  Constant3 : Constant  Value=[0;0]
  JointTorqueDes_Nm : Outport  InitialOutput=[0;0]
  wires:
  Constant3/1 -> JointTorqueDes_Nm/1

== system LibraryFM/Controller_AFFC/run ==
  q_ref_in : Inport
  qdot_ref_in : Inport  Port=2
  qddot_ref_in : Inport  Port=3
  Action Port : ActionPort  InitializeStates=reset
  q_ref : Outport  InitialOutput=[0;0]
  qdot_ref : Outport  Port=2  InitialOutput=[0;0]
  qddot_ref : Outport  Port=3  InitialOutput=[0;0]
  wires:
  q_ref_in/1 -> q_ref/1
  qddot_ref_in/1 -> qddot_ref/1
  qdot_ref_in/1 -> qdot_ref/1

== system LibraryFM/Controller_PD/PD + nonlin ==
  q_ref : Inport
  qdot_ref : Inport  Port=2
  qddot_ref : Inport  Port=3
  RobotBus : Inport  Port=4
  systemState : Inport  Port=5
  B(q) : MATLAB Function  TreatAsAtomicUnit=on
  Bus Creator : BusCreator  Inputs=5
  Bus Selector : BusSelector  OutputSignals=qJointSpace.q,qJointSpace.qdot
  Compare To Constant : simulink/Logic and Bit Operations/Compare To Constant  relop===  const=4  OutDataTypeStr=boolean
  DesiredTorque_PID : Display
  Kd : Gain  Gain=0.1
  Kp : Gain  Gain=2
  Sum : Sum  Inputs=|+-
  Sum1 : Sum  Inputs=|++
  Sum2 : Sum  Inputs=|+-
  Sum3 : Sum  Inputs=+++
  Terminator : Terminator
  nonlinear compensation : MATLAB Function  TreatAsAtomicUnit=on
  JointTorqueDes_Nm : Outport
  ToLogger : Outport  Port=2
  wires:
  Bus Creator/1 -> ToLogger/1  "ToLoggerPD"
  Compare To Constant/1 -> Terminator/1
  systemState/1 -> Compare To Constant/1
  qddot_ref/1 -> Sum3/3, Bus Creator/5  "qddot_ref"
  RobotBus/1 -> Bus Selector/1
  Sum1/1 -> DesiredTorque_PID/1, JointTorqueDes_Nm/1
  Sum2/1 -> Kd/1  "e_d"
  qdot_ref/1 -> Sum2/1, Bus Creator/4  "qdot_ref"
  Sum/1 -> Kp/1  "e_p"
  q_ref/1 -> Sum/1, Bus Creator/3  "q_ref"
  Bus Selector/1 -> B(q)/2(q), nonlinear compensation/1(q), Sum/2  "<q>"
  Bus Selector/2 -> Sum2/2, nonlinear compensation/2(qdot)  "<qdot>"
  Kp/1 -> Sum3/1
  Kd/1 -> Sum3/2
  Sum3/1 -> B(q)/1(y)
  B(q)/1(tau) -> Bus Creator/1, Sum1/1  "tau_y"
  nonlinear compensation/1(tau) -> Bus Creator/2, Sum1/2  "tau_nlcomp"

== system LibraryFM/Controller_PD/default ==
  Action Port : ActionPort  InitializeStates=reset
  Constant3 : Constant  Value=[0;0]
  JointTorqueDes_Nm : Outport  InitialOutput=[0;0]
  wires:
  Constant3/1 -> JointTorqueDes_Nm/1

== system LibraryFM/Controller_PD/homing - active ==
  note: The velocity and acceleration references are set to [0;0] for stability.
  note: These blocks hold the first sample of the input
      | when the block is enabled (through the action port)
  HomePosition : Inport
  RobotBus : Inport  Port=2
  Action Port : ActionPort  InitializeStates=reset
  Bus Selector : BusSelector  OutputSignals=qJointSpace.q
  Constant1 : Constant
  Constant2 : Constant  Value=[0;0]
  Constant4 : Constant  Value=[0;0]
  Counter Free-Running : simulink/Sources/Counter Free-Running  NumBits=32  tsamp=-1
  CrossFade : VariousBlocksLibrary/Various/CrossFade
  Cycloid : VariousBlocksLibrary/Various/Cycloid
  Manual Switch : ManualSwitch  CurrentSetting=0
  Memory1 : Memory
  Rate Limiter : RateLimiter  RisingSlewLimit=0.1  FallingSlewLimit=-0.2  SampleTimeMode=inherited
  Switch : Switch  Threshold=1
  q_ref : Outport  InitialOutput=[0;0]
  qdot_ref : Outport  Port=2  InitialOutput=[0;0]
  qddot_ref : Outport  Port=3  InitialOutput=[0;0]
  wires:
  Constant4/1 -> qddot_ref/1
  CrossFade/1 -> q_ref/1
  Manual Switch/1 -> CrossFade/1
  Memory1/1 -> Switch/1
  Counter Free-Running/1 -> Switch/2
  Switch/1 -> Manual Switch/1, Memory1/1
  Constant1/1 -> Rate Limiter/1
  Rate Limiter/1 -> Cycloid/1
  Cycloid/1 -> CrossFade/3
  HomePosition/1 -> CrossFade/2
  RobotBus/1 -> Bus Selector/1
  Bus Selector/1 -> Switch/3, Manual Switch/2  "<q>"
  Constant2/1 -> qdot_ref/1

== system LibraryFM/Controller_PD/homing - done ==
  Action Port : ActionPort
  Constant : Constant  Value=[0;0]
  JointTorqueDes_Nm : Outport  InitialOutput=[0;0]
  wires:
  Constant/1 -> JointTorqueDes_Nm/1

== system LibraryFM/Controller_PD/idle (no torque) ==
  Action Port : ActionPort  InitializeStates=reset
  Constant3 : Constant  Value=[0;0]
  JointTorqueDes_Nm : Outport  InitialOutput=[0;0]
  wires:
  Constant3/1 -> JointTorqueDes_Nm/1

== system LibraryFM/Controller_PD/run ==
  q_ref_in : Inport
  qdot_ref_in : Inport  Port=2
  qddot_ref_in : Inport  Port=3
  Action Port : ActionPort  InitializeStates=reset
  q_ref : Outport  InitialOutput=[0;0]
  qdot_ref : Outport  Port=2  InitialOutput=[0;0]
  qddot_ref : Outport  Port=3  InitialOutput=[0;0]
  wires:
  q_ref_in/1 -> q_ref/1
  qddot_ref_in/1 -> qddot_ref/1
  qdot_ref_in/1 -> qdot_ref/1

== system LibraryFM/DataFromEtherCAT/Calculate Arrange Joint and Op Space ==
  note: Here all angles of the parallel mechanism are calculated
      | based on the endpoint position, though this may still lead to incorrect
      | estimations of the internal angles (e.g. it is possible that on of the elbows
      | has gone through a singular position already). So perhaps I should also include
      | a different way of calculating the internal angles
  BusActuators : Inport
  Bus Creator1 : BusCreator  Inputs=3
  Bus Creator2 : BusCreator  Inputs=3
  Bus Selector2 : BusSelector  OutputSignals=BusActuator1.JointPosition_rad,BusActuator2.JointPosition_rad,BusActuator1.JointVelocity_rads,BusActuator2.JointVelocity_rads
  Display : Display
  Gain : Gain  Gain=180/pi
  Ground : Ground
  IK all joints : MATLAB Function  TreatAsAtomicUnit=on
  Mux : Mux  Inputs=2
  Mux1 : Mux  Inputs=2
  Terminator1 : Terminator
  Terminator2 : Terminator
  forward kinematics : Subsystem
  xOpSpace : Outport
  qJointSpace : Outport  Port=2
  wires:
  Gain/1 -> Display/1
  IK all joints/1(q_all) -> Bus Creator2/3  "q_all"
  Mux/1 -> Bus Creator2/1, Gain/1, forward kinematics/1(JointPosition_rad)  "q"
  Mux1/1 -> Bus Creator2/2, forward kinematics/2(JointVelocity_rads)  "qdot"
  Bus Selector2/4 -> Mux1/2  "<JointVelocity_rads>"
  Bus Selector2/3 -> Mux1/1  "<JointVelocity_rads>"
  Bus Selector2/2 -> Mux/2  "<JointPosition_rad>"
  Bus Selector2/1 -> Mux/1  "<JointPosition_rad>"
  BusActuators/1 -> Bus Selector2/1
  Bus Creator2/1 -> qJointSpace/1  "qJointSpace"
  Ground/1 -> forward kinematics/3(JointAcceleration_rads2)
  forward kinematics/4(J) -> Bus Creator1/3  "jacobian"
  Bus Creator1/1 -> xOpSpace/1  "xOpSpace"
  forward kinematics/1(x) -> Bus Creator1/1, IK all joints/1(x)  "x"
  forward kinematics/2(xdot) -> Bus Creator1/2  "xdot"
  forward kinematics/3(xddot) -> Terminator1/1
  forward kinematics/5(Jdot) -> Terminator2/1

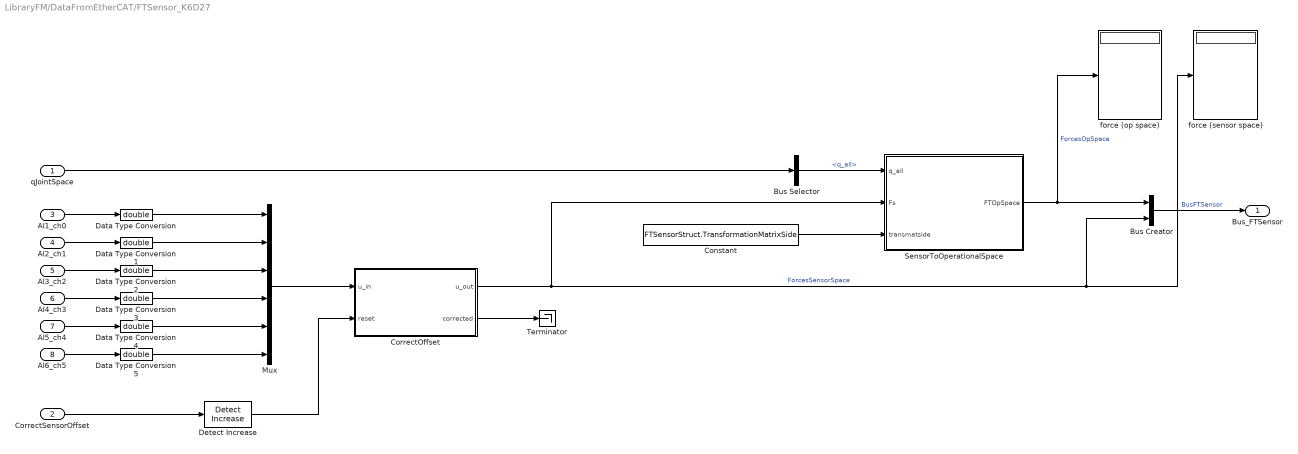
== system LibraryFM/DataFromEtherCAT/FTSensor_K6D27 ==
  qJointSpace : Inport
  CorrectSensorOffset : Inport  Port=2
  AI1_ch0 : Inport  Port=3
  AI2_ch1 : Inport  Port=4
  AI3_ch2 : Inport  Port=5
  AI4_ch3 : Inport  Port=6
  AI5_ch4 : Inport  Port=7
  AI6_ch5 : Inport  Port=8
  Bus Creator : BusCreator  Inputs=2
  Bus Selector : BusSelector  OutputSignals=q_all
  Constant : Constant  Value=FTSensorStruct.TransformationMatrixSide
  CorrectOffset : MATLAB Function  TreatAsAtomicUnit=on
  Data Type Conversion{,1..5} (6 alike) : DataTypeConversion  OutDataTypeStr=double
  Detect Increase : simulink/Logic and Bit Operations/Detect Increase  vinit=0.0  InputProcessing=Inherited  OutDataTypeStr=boolean
  Mux : Mux  Inputs=6
  SensorToOperationalSpace : MATLAB Function  TreatAsAtomicUnit=on
  Terminator : Terminator
  force (op space) : Display
  force (sensor space) : Display
  Bus_FTSensor : Outport
  wires:
  Bus Selector/1 -> SensorToOperationalSpace/1(q_all)  "<q_all>"
  qJointSpace/1 -> Bus Selector/1
  AI2_ch1/1 -> Data Type Conversion1/1
  AI1_ch0/1 -> Data Type Conversion/1
  Mux/1 -> CorrectOffset/1(u_in)
  CorrectSensorOffset/1 -> Detect Increase/1
  Detect Increase/1 -> CorrectOffset/2(reset)
  AI6_ch5/1 -> Data Type Conversion5/1
  AI5_ch4/1 -> Data Type Conversion4/1
  AI4_ch3/1 -> Data Type Conversion3/1
  AI3_ch2/1 -> Data Type Conversion2/1
  CorrectOffset/2(corrected) -> Terminator/1
  CorrectOffset/1(u_out) -> force (sensor space)/1, Bus Creator/2, SensorToOperationalSpace/2(Fs)  "ForcesSensorSpace"
  Data Type Conversion/1 -> Mux/1
  Data Type Conversion1/1 -> Mux/2
  Data Type Conversion2/1 -> Mux/3
  Data Type Conversion3/1 -> Mux/4
  Data Type Conversion4/1 -> Mux/5
  Data Type Conversion5/1 -> Mux/6
  SensorToOperationalSpace/1(FTOpSpace) -> Bus Creator/1, force (op space)/1  "ForcesOpSpace"
  Bus Creator/1 -> Bus_FTSensor/1  "BusFTSensor"
  Constant/1 -> SensorToOperationalSpace/3(transmatside)

== system LibraryFM/DataToEtherCAT/FTSensorError ==
  RobotBus : Inport
  AvoidAlgebraicLoop : Memory
  Bus Selector : BusSelector  OutputSignals=BusFTSensor.ForcesSensorSpace
  Constant : Constant  Value=RobotStruct.FTSensor.MaxAllowableForcesTorqueSensor
  CreateSingleErrorValue : LibraryFM/ToActuator1/DriveEnableLogic/CreateSingleErrorValue
  Detect Change : simulink/Logic and Bit Operations/Detect Change  vinit=0  InputProcessing=Inherited  OutDataTypeStr=boolean
  FTSensorLastError : Display
  LatchRising : LibraryFM/Utilities/LatchRising  ic=0
  MATLAB Function : MATLAB Function  TreatAsAtomicUnit=on
  ShowFTSensorErrorLatched : Display
  FTSensorError : Outport
  FTSensorErrorLatched : Outport  Port=2
  wires:
  Bus Selector/1 -> MATLAB Function/1(ForcesTorques)  "<ForcesSensorSpace>"
  RobotBus/1 -> Bus Selector/1
  Detect Change/1 -> LatchRising/Trigger
  AvoidAlgebraicLoop/1 -> FTSensorError/1, LatchRising/1, Detect Change/1
  LatchRising/1 -> FTSensorErrorLatched/1, ShowFTSensorErrorLatched/1
  CreateSingleErrorValue/1 -> AvoidAlgebraicLoop/1
  MATLAB Function/1(e) -> CreateSingleErrorValue/1, FTSensorLastError/1
  Constant/1 -> MATLAB Function/2(MaxForcesTorques)
